simulink model "parameterOptimizerExcavator"  (R2025a)
settings: Solver=ode15s  StartTime=0.0  StopTime=10  RelTol=1e-3
model workspace (MATLAB code in the model file):
  | %% Weights
  | bomWeight = 200.04;
  | stickWeight = 158.71;
  | bucketWeight = 71.311;
  | 
  | %% Cylinders
  | % cylinder One
  | cylinderOneDamping = 1000;
  | cylinderOnePistonCrossSectionalAreaChamberA = 0.1403;
  | cylinderOnePistonCrossSectionalAreaChamberB = 0.17443;
  | cylinderOnePistonStroke = 529.98;
  | cylinderOneDeadVolumeChamberA = 0.04316;
  | cylinderOneDeadVolumeChamberB = 0.054177;
  | 
  | %cylinder Two
  | cylinderTwoDamping = 1000;
  | cylinderTwoPistonCrossSectionalAreaChamberA = 0.18189;
  | cylinderTwoPistonCrossSectionalAreaChamberB = 0.1784;
  | cylinderTwoPistonStroke = 652.71;
  | cylinderTwoDeadVolumeChamberA = 0.036781;
  | cylinderTwoDeadVolumeChamberB = 0.054436;
  | 
  | %% Input
  | inputDelay = 2;
  | 
  | %% Pump
  | %pumpDisplayment = 18;
  | 
  | PGV1 = 0;
  | PGV2 = 10.37811;
  | PGV3 = 21.47722;
  | PGV4 = 32.57634;
  | PGV5 = 43.67545;
  | PGV6 = 54.77457;
  | PGV7 = 65.87369;
  | PGV8 = 76.9728;
  | PGV9 = 88.07192;
  | PGV10 = 99.17103;
  | PGV11 = 110.27015;
  | PGV12 = 121.36926;
  | PGV13 = 132.46838;
  | PGV14 = 143.56749;
  | PGV15 = 154.66661;
  | PGV16 = 165.76572;
  | PGV17 = 176.86484;
  | PGV18 = 187.96396;
  | PGV19 = 199.06307;
  | PGV20 = 210.16219;
  | PGV21 = 221.2613;
  | PGV22 = 232.36042;
  | PGV23 = 243.45953;
  | PGV24 = 254.55865;
  | PGV25 = 265.65776;
  | PGV26 = 276.75688;
  | PGV27 = 287.85599;
  | PGV28 = 298.95511;
  | PGV29 = 310.05422;
  | PGV30 = 321.15334;
  | pumpPressureGainVector = [PGV1 PGV2 PGV3 PGV4 PGV5 PGV6 PGV7 PGV8 PGV9 PGV10 PGV11 PGV12 PGV13 PGV14 PGV15 PGV16 PGV17 PGV18 PGV19 PGV20 PGV21 PGV22 PGV23 PGV24 PGV25 PGV26 PGV27 PGV28 PGV29 PGV30];
  | 
  | SAV1 = 1000;
  | SAV2 = 1200;
  | SAV3 = 1500;
  | SAV4 = 1800;
  | pumpAnglularVelocityVector = [SAV1 SAV2 SAV3 SAV4];
  | 
  | pumpAngluarVelocityThreshold = 10;
  | 
  | %% new pump
  | pumpDisplacement = 0.00013254;
  | pumpNominalShaftAngularVelocity = 116.48;
  | pumpNominalPressureGain = 4.2749;
undefined symbols (not defined in the file): Excavator_Param, X, Y, Z
libraries: sm_lib x65, fl_lib x19, nesl_utility x17, SimscapeFluids_lib x9, simulink_extras x8
(part 1 of 4)
settings Model: Creator=eliasalbag  LastModifiedBy=Viktor Traktor
settings DataIOCC: ReturnWorkspaceOutputsName=SDOSimTest_Log

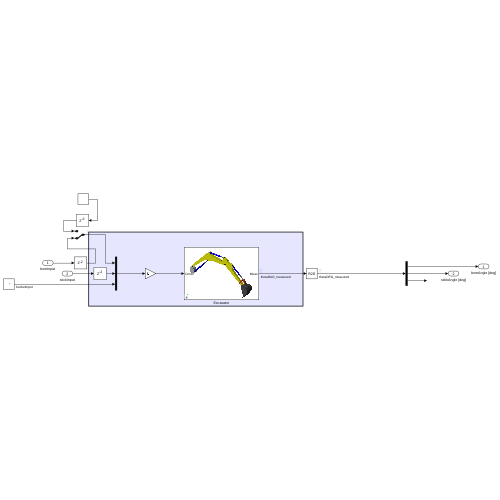
[thumbnail: Simulink's stored preview of the top-level diagram]
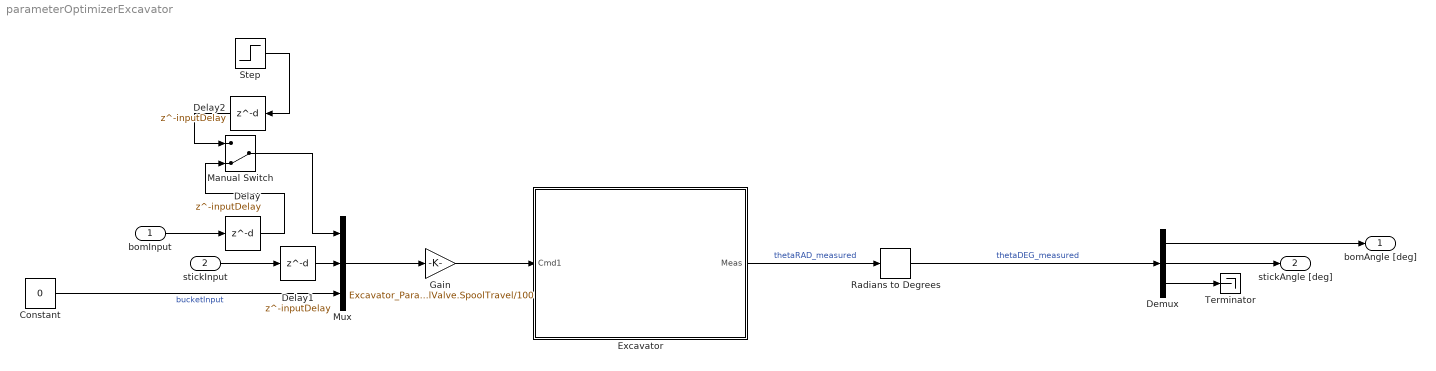
== system parameterOptimizerExcavator ==
  bomInput : Inport
  stickInput : Inport  Port=2
  Constant : Constant  Value=0
  Delay : Delay  DelayLength=inputDelay
  Delay1 : Delay  DelayLength=inputDelay
  Delay2 : Delay  DelayLength=inputDelay
  Demux : Demux  Outputs=3
  Excavator : Subsystem  mask{D=0}
      mask prompts: D "Damping"
      mask Display: image('Skärmbild 2025-05-16 122333.png');
  Gain : Gain  Gain=Excavator_Param.DirectionalValve.SpoolTravel/100
  Manual Switch : ManualSwitch  CurrentSetting=0
  Mux : Mux  Inputs=3
  Radians to Degrees : simulink_extras/Transformations/Radians to Degrees
  Step : Step  After=-100  SampleTime=0.01
  Terminator : Terminator
  bomAngle [deg] : Outport
  stickAngle [deg] : Outport  Port=2
  wires:
  Excavator/1(Meas) -> Radians to Degrees/1  "thetaRAD_measured"
  Mux/1 -> Gain/1
  bomInput/1 -> Delay/1
  Radians to Degrees/1 -> Demux/1  "thetaDEG_measured"
  Constant/1 -> Mux/3  "bucketInput"
  Demux/3 -> Terminator/1
  Demux/2 -> stickAngle [deg]/1
  Demux/1 -> bomAngle [deg]/1
  Gain/1 -> Excavator/1(Cmd1)
  stickInput/1 -> Delay1/1
  Delay/1 -> Manual Switch/2
  Delay1/1 -> Mux/2
  Manual Switch/1 -> Mux/1
  Step/1 -> Delay2/1
  Delay2/1 -> Manual Switch/1

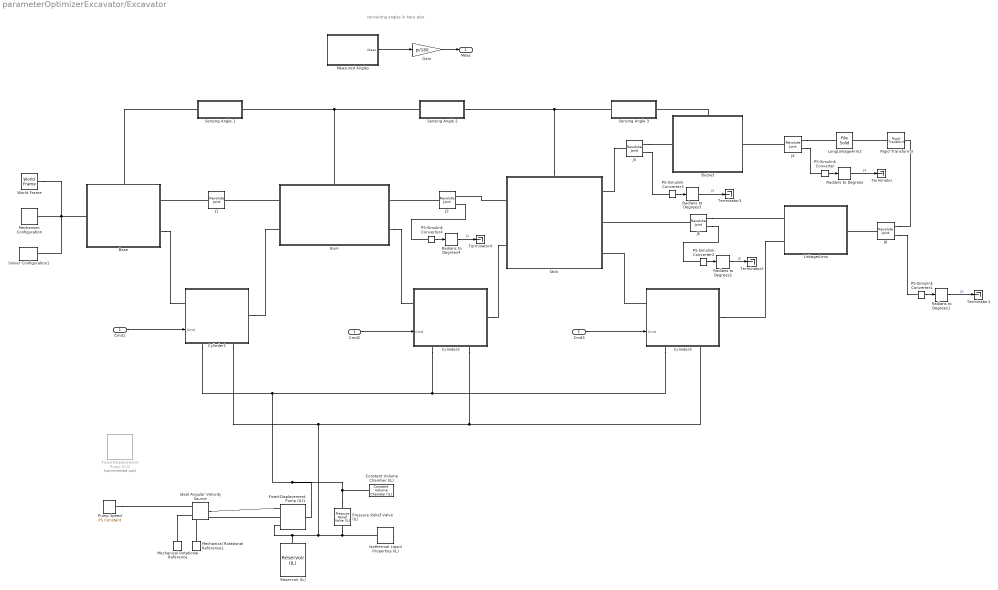
== system parameterOptimizerExcavator/Excavator ==
  note: converting angles in here also
  Cmd1 : Inport
  Base : Subsystem
      settings: PortSchema="{\"entries\":[{\"content\":{\"sides\":[{\"content\":{\"connectorIds\":[\"LConn1\"]},\"type\":\"ConnectorPlacement.EquallySpacedRectSide\",\"uuid\":\"40ecd481-0f87-4ac6-81e7-411d2e7a87dc\"},{\"content\":{\"connectorIds\":[\"RConn1\",\"RConn2\"],\"side\":\"RIGHT\"},\"type\":\"ConnectorPlacement.EquallySpacedRectSide\",\"uuid\":\"4ae56660-704d-4a11-a2e7-42dc450a906f\"},{\"content\":{\"connectorIds\":[\"LConn2\"],\"side\":\"TOP\"},\"type\":\"ConnectorPlacement.EquallySpacedRectSide\",\"uuid\":\"88ba4c47-909e-475c-98b2-d2ec55f2c628\"}]},\"type\":\"ConnectorPlacement.EquallySpacedConnector\",\"uuid\":\"875afadf-353a-4577-a20f-50c01c00738f\"}],\"packageUris\":[\"http://schema.mathworks.com/mf0/Connector/R2020b\"],\"version\":\"1.0\"}"
      mask Display: image('Skärmbild 2025-04-30 163637.png');
  Bom : Subsystem
      settings: PortSchema="{\"entries\":[{\"content\":{\"sides\":[{\"content\":{\"connectorIds\":[\"LConn1\",\"LConn2\"]},\"type\":\"ConnectorPlacement.EquallySpacedRectSide\",\"uuid\":\"7ad98941-c155-4b77-821c-441aa02f495c\"},{\"content\":{\"connectorIds\":[\"RConn1\",\"RConn2\"],\"side\":\"RIGHT\"},\"type\":\"ConnectorPlacement.EquallySpacedRectSide\",\"uuid\":\"f5fb3b40-b535-47bd-a749-2c1f436a2cdb\"},{\"content\":{\"connectorIds\":[\"LConn3\"],\"side\":\"TOP\"},\"type\":\"ConnectorPlacement.EquallySpacedRectSide\",\"uuid\":\"726e9b82-bc1f-498c-98b8-155d9f00309d\"}]},\"type\":\"ConnectorPlacement.EquallySpacedConnector\",\"uuid\":\"e0155be9-0ff1-4a5f-ae8d-a122aa83cbac\"}],\"packageUris\":[\"http://schema.mathworks.com/mf0/Connector/R2020b\"],\"version\":\"1.0\"}"
      mask Display: image('Skärmbild 2025-05-01 094232.png');
  Bucket : Subsystem
      settings: PortSchema="{\"entries\":[{\"content\":{\"sides\":[{\"content\":{\"connectorIds\":[\"LConn1\"]},\"type\":\"ConnectorPlacement.EquallySpacedRectSide\",\"uuid\":\"5de28302-4101-44f3-9c23-279c450fdd15\"},{\"content\":{\"connectorIds\":[\"RConn1\"],\"side\":\"RIGHT\"},\"type\":\"ConnectorPlacement.EquallySpacedRectSide\",\"uuid\":\"b0db8830-510e-47ef-9140-b2643c0c8376\"},{\"content\":{\"connectorIds\":[\"LConn2\"],\"side\":\"TOP\"},\"type\":\"ConnectorPlacement.EquallySpacedRectSide\",\"uuid\":\"09d89f5e-8f1e-4430-8208-03f2526c5b85\"}]},\"type\":\"ConnectorPlacement.EquallySpacedConnector\",\"uuid\":\"9e049277-2e17-4388-a3ed-55a7f1fde4cc\"}],\"packageUris\":[\"http://schema.mathworks.com/mf0/Connector/R2020b\"],\"version\":\"1.0\"}"
      mask Display: image('Skärmbild 2025-05-02 202436.png');
  Cmd2 : InportShadow
  Cmd3 : InportShadow
  Constant Volume Chamber (IL) : fl_lib/Isothermal Liquid/Elements/Constant Volume Chamber (IL)  volume=1e-4 m^3  p_I_specify=off  p_I_priority=High  p_I=0.101325 MPa  p_I_nominal_specify=off  p_I_nominal_value=1  p_I_nominal_unit=MPa
      settings: InternalSimscapePortConfiguration="{\"Bottom\":[],\"Left\":[{\"id\":\"A\",\"label\":\"A\",\"type\":\"foundation.isothermal_liquid.isothermal_liquid\"}],\"Right\":[],\"Top\":[]}"
  Cylinder1 : Subsystem
      settings: PortSchema="{\"entries\":[{\"content\":{\"sides\":[{\"content\":{\"connectorIds\":[\"LConn1\",\"In1\"]},\"type\":\"ConnectorPlacement.EquallySpacedRectSide\",\"uuid\":\"958c3393-df8d-4c6f-89df-92ae8f6a338c\"},{\"content\":{\"connectorIds\":[\"RConn1\"],\"side\":\"RIGHT\"},\"type\":\"ConnectorPlacement.EquallySpacedRectSide\",\"uuid\":\"7fbd6d33-fc32-41eb-a764-fc12f800bd43\"},{\"content\":{\"side\":\"TOP\"},\"type\":\"ConnectorPlacement.EquallySpacedRectSide\",\"uuid\":\"2a2fac5b-7b8e-4bd5-9693-24b32f9ec475\"},{\"content\":{\"connectorIds\":[\"RConn2\",\"RConn3\"],\"side\":\"BOTTOM\"},\"type\":\"ConnectorPlacement.EquallySpacedRectSide\",\"uuid\":\"152fac46-1909-43ca-b282-7d5220c5a160\"}]},\"type\":\"ConnectorPlacement.EquallySpacedConnector\",\"uuid\":\"942b4f77-d0ef-4ef4-96e1-eaf5fcd20a12\"}],\"packageUris\":[\"http://schema.mathworks.com/mf0/Connector/R2020b\"],\"version\":\"1.0\"}"
      mask Display: image('Skärmbild 2025-05-02 202508.png');
  Cylinder2 : Subsystem
      settings: PortSchema="{\"entries\":[{\"content\":{\"sides\":[{\"content\":{\"connectorIds\":[\"LConn1\",\"In1\"]},\"type\":\"ConnectorPlacement.EquallySpacedRectSide\",\"uuid\":\"57f8ce67-ce53-4554-827a-ade4073837f1\"},{\"content\":{\"connectorIds\":[\"RConn1\"],\"side\":\"RIGHT\"},\"type\":\"ConnectorPlacement.EquallySpacedRectSide\",\"uuid\":\"2d7b50e6-8862-4672-bf86-700cfda39af2\"},{\"content\":{\"side\":\"TOP\"},\"type\":\"ConnectorPlacement.EquallySpacedRectSide\",\"uuid\":\"6448b736-3558-4b72-a3be-02cdc9d0d1c5\"},{\"content\":{\"connectorIds\":[\"RConn2\",\"RConn3\"],\"side\":\"BOTTOM\"},\"type\":\"ConnectorPlacement.EquallySpacedRectSide\",\"uuid\":\"d65b4c05-b673-4eae-8b65-2a19aca8236c\"}]},\"type\":\"ConnectorPlacement.EquallySpacedConnector\",\"uuid\":\"43cefb1d-1bfc-4d29-867b-e7529d2d57fb\"}],\"packageUris\":[\"http://schema.mathworks.com/mf0/Connector/R2020b\"],\"version\":\"1.0\"}"
      mask Display: image('Skärmbild 2025-05-02 202508.png');
  Cylinder3 : Subsystem
      settings: PortSchema="{\"entries\":[{\"content\":{\"sides\":[{\"content\":{\"connectorIds\":[\"LConn1\",\"In1\"]},\"type\":\"ConnectorPlacement.EquallySpacedRectSide\",\"uuid\":\"57f8ce67-ce53-4554-827a-ade4073837f1\"},{\"content\":{\"connectorIds\":[\"RConn1\"],\"side\":\"RIGHT\"},\"type\":\"ConnectorPlacement.EquallySpacedRectSide\",\"uuid\":\"2d7b50e6-8862-4672-bf86-700cfda39af2\"},{\"content\":{\"side\":\"TOP\"},\"type\":\"ConnectorPlacement.EquallySpacedRectSide\",\"uuid\":\"6448b736-3558-4b72-a3be-02cdc9d0d1c5\"},{\"content\":{\"connectorIds\":[\"RConn2\",\"RConn3\"],\"side\":\"BOTTOM\"},\"type\":\"ConnectorPlacement.EquallySpacedRectSide\",\"uuid\":\"3b9bbe70-3b78-4081-87f5-0faddfe5faea\"}]},\"type\":\"ConnectorPlacement.EquallySpacedConnector\",\"uuid\":\"43cefb1d-1bfc-4d29-867b-e7529d2d57fb\"}],\"packageUris\":[\"http://schema.mathworks.com/mf0/Connector/R2020b\"],\"version\":\"1.0\"}"
      mask Display: image('Skärmbild 2025-05-02 202508.png');
  Fixed-Displacement Pump (IL)1 : SimscapeFluids_lib/Isothermal Liquid/Pumps & Motors/Fixed-Displacement Pump (IL)  leakage_friction_spec=fluids.isothermal_liquid.pumps_motors.enum.pump_motor_loss_spec.analytical  displacement=pumpDisplacement m^3/rad  omega_nominal=pumpNominalShaftAngularVelocity rad/s  p_nominal=pumpNominalPressureGain MPa  vol_eff_nominal=0.92  mech_eff_nominal=0.88  no_load_torque=0 N*m  p_diff_eff_TLU=[.1, 1, 2] MPa  omega_eff_TLU=[250, 500, 1000, 2000, 3000, 4000] rpm  vol_eff_TLU=[.816, .908, .954, .977, .981, .984; .325, .663, .831, .916, .925, .946; .137, .568, .78, .892, .893, .91]  mech_eff_TLU=[.996, .996, .996, .996, .996, .996; .988, .989, .989, .989, .989, .99; .981, .981, .982, .982, .983, .984]  p_diff_loss_TLU=[.1, 1, 2] MPa  omega_loss_TLU=[250, 500, 1000, 2000, 3000, 4000] rpm  vol_loss_TLU=1e-3 * [.023, .023, .023, .023, .0285, .032; .0844, .0842, .0845, .084, .1125, .108; .1079, .108, .11, .108, .1605, .18] m^3/s  mech_loss_TLU=[.002, .002, .002, .002, .002, .002; .0607, .0556, .0556, .0556, .0556, .0505; .1937, .1937, .1833, .1833, .1729, .1626] N*m  vol_eff_min=1e-3  vol_eff_max=1  mech_eff_min=1e-3  mech_eff_max=1  pressure_threshold=1e-3 MPa  omega_threshold=100 rpm  supplied_range_check=simscape.enum.assert.action.none  pump_mode_check=simscape.enum.assert.action.none  pressure_check=simscape.enum.assert.action.none  p_min_valid=0.101325 MPa
      settings: InternalSimscapePortConfiguration="{\"Bottom\":[{\"id\":\"A\",\"label\":\"A\",\"type\":\"foundation.isothermal_liquid.isothermal_liquid\"}],\"Left\":[],\"Right\":[{\"id\":\"R\",\"label\":\"R\",\"type\":\"foundation.mechanical.rotational.rotational\"},{\"id\":\"C\",\"label\":\"C\",\"type\":\"foundation.mechanical.rotational.rotational\"}],\"Top\":[{\"id\":\"B\",\"label\":\"B\",\"type\":\"foundation.isothermal_liquid.isothermal_liquid\"}]}"
  Fixed-Displacement Pump (IL)2 : SimscapeFluids_lib/Isothermal Liquid/Pumps & Motors/Fixed-Displacement Pump (IL)  Commented=on  PartSpecification="{\"CollectionId\":\"SimscapeFluids\",\"CollectionVersion\":\"1.0.0\",\"DatasetId\":\"Eaton|PVM:018|simscape.fluids.isothermalLiquid.fixedDisplacementPump\",\"DisplayName\":\"Eaton:PVM:018\"}"  leakage_friction_spec=fluids.isothermal_liquid.pumps_motors.enum.pump_motor_loss_spec.table_efficiency  displacement=pumpDisplayment cm^3/rev  omega_nominal=1800 % Parameter not set rpm  p_nominal=10 % Parameter not set MPa  vol_eff_nominal=0.92 % Parameter not set  mech_eff_nominal=0.88 % Parameter not set  no_load_torque=0 % Parameter not set N*m  p_diff_eff_TLU=pumpPressureGainVector bar  omega_eff_TLU=pumpAnglularVelocityVector rpm  vol_eff_TLU=[0.9933773 0.9986255 1 1;0.9908815 0.9970227 0.9988015 0.9986391;0.9882123 0.9953086 0.9972361 0.9971836;0.9855432 0.9935944 0.9956708 0.9957282;0.982874 0.9918803 0.9941054 0.9942727;0.9809628 0.9901046 0.9924794 0.992827;0.9800522 0.9882469 0.9908036 0.991394;0.9791415 0.9863891 0.9891279 0.989961;0.9782309 0.9845314 0.9874521 0.988528;0.9773202 0.9826736 0.9857764 0.987095;0.9763834 0.9808159 0.984196 0.9858236;0.9754406 0.9789581 0.9826224 0.9845647;0.9744978 0.9771004 0.9810489 0.9833058;0.973555 0.9752426 0.9794753 0.9820468;0.9722953 0.9733813 0.9778456 0.9807183;0.9704577 0.9715138 0.9761613 0.9792853;0.9686202 0.9696463 0.9744771 0.9778523;0.9667827 0.9677789 0.9727928 0.9764193;0.9649452 0.9659114 0.9711086 0.9749863;0.9633236 0.9640355 0.9698474 0.9737089;0.9617784 0.9621582 0.9686255 0.97245;0.9602331 0.9602809 0.9674035 0.9711911;0.9586878 0.9584036 0.9661816 0.9699321;0.9563057 0.9564651 0.9651295 0.9682414;0.9524066 0.9544264 0.9642731 0.9658002;0.9485075 0.9523877 0.9634167 0.9633591;0.9446085 0.950349 0.9625603 0.9609179;0.9407094 0.9483103 0.9617039 0.9584767;0.9360576 0.9469113 0.9607892 0.9566098;0.931177 0.9456055 0.9598677 0.9548364] % Datasheet derived  mech_eff_TLU=[0.001 0.001 0.01192 0.001;0.54982 0.55826 0.52817 0.51523;0.7457 0.73749 0.72894 0.7104;0.82552 0.81697 0.8091 0.79478;0.86515 0.8517 0.84128 0.83826;0.89161 0.87592 0.86458 0.86826;0.89855 0.8853 0.87936 0.88694;0.9055 0.89471 0.89419 0.90566;0.91246 0.90416 0.90907 0.91532;0.91943 0.91365 0.91743 0.92476;0.92432 0.92008 0.92338 0.92926;0.92874 0.9261 0.92933 0.93321;0.93316 0.93215 0.9353 0.93716;0.93759 0.93822 0.94128 0.94113;0.94083 0.94329 0.94509 0.94404;0.94196 0.94674 0.94701 0.94533;0.94308 0.9502 0.94893 0.94662;0.94421 0.95368 0.95086 0.94792;0.94534 0.95717 0.9528 0.94922;0.94547 0.95801 0.95262 0.94983;0.94521 0.95819 0.95216 0.95032;0.94494 0.95838 0.9517 0.95082;0.94468 0.95857 0.95124 0.95132;0.94485 0.95778 0.9502 0.95201;0.94566 0.95552 0.9485 0.95304;0.9444 0.95324 0.94681 0.95407;0.94245 0.95096 0.94511 0.9551;0.9405 0.94866 0.94341 0.95614;0.94063 0.94494 0.94137 0.95543;0.94151 0.941 0.93927 0.95443] % Datasheet derived  p_diff_loss_TLU=[.1, 1, 2] % Parameter not set MPa  omega_loss_TLU=[250, 500, 1000, 2000, 3000, 4000] % Parameter not set rpm  vol_loss_TLU=1e-3 * [.023, .023, .023, .023, .0285, .032; .0844, .0842, .0845, .084, .1125, .108; .1079, .108, .11, .108, .1605, .18] % Parameter not set m^3/s  mech_loss_TLU=[.002, .002, .002, .002, .002, .002; .0607, .0556, .0556, .0556, .0556, .0505; .1937, .1937, .1833, .1833, .1729, .1626] % Parameter not set N*m  vol_eff_min=1e-3 % Parameter not set  vol_eff_max=1 % Parameter not set  mech_eff_min=1e-3 % Parameter not set  mech_eff_max=1 % Parameter not set  pressure_threshold=0.001 % Library default MPa  omega_threshold=pumpAngluarVelocityThreshold rpm  supplied_range_check=simscape.enum.assert.action.none  pump_mode_check=simscape.enum.assert.action.none  pressure_check=simscape.enum.assert.action.none  p_min_valid=0.101325 % Parameter not set MPa
      settings: AttributesFormatString=Eaton:PVM:018  InternalSimscapePortConfiguration="{\"Bottom\":[{\"id\":\"A\",\"label\":\"A\",\"type\":\"foundation.isothermal_liquid.isothermal_liquid\"}],\"Left\":[],\"Right\":[{\"id\":\"R\",\"label\":\"R\",\"type\":\"foundation.mechanical.rotational.rotational\"},{\"id\":\"C\",\"label\":\"C\",\"type\":\"foundation.mechanical.rotational.rotational\"}],\"Top\":[{\"id\":\"B\",\"label\":\"B\",\"type\":\"foundation.isothermal_liquid.isothermal_liquid\"}]}"
  Gain : Gain  Gain=pi/180
  Ideal Angular Velocity Source : fl_lib/Mechanical/Mechanical Sources/Ideal Angular Velocity Source
  Isothermal Liquid Properties (IL) : fl_lib/Isothermal Liquid/Utilities/Isothermal Liquid Properties (IL)  rho_L_atm=845 kg/m^3  bulk_modulus_model=foundation.enum.bulk_modulus_model.const  beta_gain=6  beta_L_atm=1.59e9 Pa  nu_atm=52.63 cSt  p_atm=0.101325 MPa  p_min=1 Pa  properties_range_check=simscape.enum.assert.action.error  air_fraction=0.004  polytropic_index=1.0  rho_g_atm=1.225 kg/m^3  air_dissolution_model=false  p_crit=3 MPa
  J1 : sm_lib/Joints/Revolute Joint  JointMode=Normal  CompositeWrenchDir=FollowerOnBase  CompositeWrenchFrame=BaseFrame  SenseConstraintForce=off  SenseConstraintTorque=off  SenseTotalForce=off  SenseTotalTorque=off  PositionTargetSpecify=on  PositionTargetPriority=Low  PositionTargetValue=0  PositionTargetValueUnits=deg  VelocityTargetSpecify=off  VelocityTargetPriority=High  VelocityTargetValue=0  VelocityTargetValueUnits=deg/s  EquilibriumPosition=0  EquilibriumPositionUnits=deg  SpringStiffness=0  SpringStiffnessUnits=N*m/deg  DampingCoefficient=Excavator_Param.Joint1.Damping  DampingCoefficientUnits=N*m/(deg/s)  LowerLimitSpecify=off  LowerLimitBound=-15  LowerLimitBoundUnits=deg  LowerLimitStiffness=1e5  LowerLimitStiffnessUnits=N*m/deg  LowerLimitDamping=10  LowerLimitDampingUnits=N*m/(deg/s)  LowerLimitTransitionRegionWidth=1  LowerLimitTransitionRegionWidthUnits=deg  UpperLimitSpecify=off  UpperLimitBound=15  UpperLimitBoundUnits=deg  UpperLimitStiffness=1e5  UpperLimitStiffnessUnits=N*m/deg  UpperLimitDamping=10  UpperLimitDampingUnits=N*m/(deg/s)  UpperLimitTransitionRegionWidth=1  UpperLimitTransitionRegionWidthUnits=deg  TorqueActuationMode=NoTorque  MotionActuationMode=ComputedMotion  SensePosition=off  SenseVelocity=off  SenseAcceleration=off  SenseTorqueForce=off  SenseLowerLimitTorqueForce=off  SenseUpperLimitTorqueForce=off
  J2 : sm_lib/Joints/Revolute Joint  JointMode=Normal  CompositeWrenchDir=FollowerOnBase  CompositeWrenchFrame=BaseFrame  SenseConstraintForce=off  SenseConstraintTorque=off  SenseTotalForce=off  SenseTotalTorque=off  PositionTargetSpecify=on  PositionTargetPriority=Low  PositionTargetValue=0  PositionTargetValueUnits=deg  VelocityTargetSpecify=off  VelocityTargetPriority=High  VelocityTargetValue=0  VelocityTargetValueUnits=deg/s  EquilibriumPosition=0  EquilibriumPositionUnits=deg  SpringStiffness=0  SpringStiffnessUnits=N*m/deg  DampingCoefficient=Excavator_Param.Joint2.Damping  DampingCoefficientUnits=N*m/(deg/s)  LowerLimitSpecify=off  LowerLimitBound=-90  LowerLimitBoundUnits=deg  LowerLimitStiffness=1e4  LowerLimitStiffnessUnits=N*m/deg  LowerLimitDamping=10  LowerLimitDampingUnits=N*m/(deg/s)  LowerLimitTransitionRegionWidth=0.1  LowerLimitTransitionRegionWidthUnits=deg  UpperLimitSpecify=on  UpperLimitBound=26  UpperLimitBoundUnits=deg  UpperLimitStiffness=1e20  UpperLimitStiffnessUnits=N*m/deg  UpperLimitDamping=1e12  UpperLimitDampingUnits=N*m/(deg/s)  UpperLimitTransitionRegionWidth=0.1  UpperLimitTransitionRegionWidthUnits=deg  TorqueActuationMode=NoTorque  MotionActuationMode=ComputedMotion  SensePosition=on  SenseVelocity=off  SenseAcceleration=off  SenseTorqueForce=off  SenseLowerLimitTorqueForce=off  SenseUpperLimitTorqueForce=off
  J3 : sm_lib/Joints/Revolute Joint  JointMode=Normal  CompositeWrenchDir=FollowerOnBase  CompositeWrenchFrame=BaseFrame  SenseConstraintForce=off  SenseConstraintTorque=off  SenseTotalForce=off  SenseTotalTorque=off  PositionTargetSpecify=off  PositionTargetPriority=High  PositionTargetValue=0  PositionTargetValueUnits=deg  VelocityTargetSpecify=off  VelocityTargetPriority=High  VelocityTargetValue=0  VelocityTargetValueUnits=deg/s  EquilibriumPosition=0  EquilibriumPositionUnits=deg  SpringStiffness=0  SpringStiffnessUnits=N*m/deg  DampingCoefficient=100  DampingCoefficientUnits=N*m/(deg/s)  LowerLimitSpecify=off  LowerLimitBound=-90  LowerLimitBoundUnits=deg  LowerLimitStiffness=1e4  LowerLimitStiffnessUnits=N*m/deg  LowerLimitDamping=10  LowerLimitDampingUnits=N*m/(deg/s)  LowerLimitTransitionRegionWidth=0.1  LowerLimitTransitionRegionWidthUnits=deg  UpperLimitSpecify=off  UpperLimitBound=90  UpperLimitBoundUnits=deg  UpperLimitStiffness=1e4  UpperLimitStiffnessUnits=N*m/deg  UpperLimitDamping=10  UpperLimitDampingUnits=N*m/(deg/s)  UpperLimitTransitionRegionWidth=0.1  UpperLimitTransitionRegionWidthUnits=deg  TorqueActuationMode=NoTorque  MotionActuationMode=ComputedMotion  SensePosition=on  SenseVelocity=off  SenseAcceleration=off  SenseTorqueForce=off  SenseLowerLimitTorqueForce=off  SenseUpperLimitTorqueForce=off
  J4 : sm_lib/Joints/Revolute Joint  JointMode=Normal  CompositeWrenchDir=FollowerOnBase  CompositeWrenchFrame=BaseFrame  SenseConstraintForce=off  SenseConstraintTorque=off  SenseTotalForce=off  SenseTotalTorque=off  PositionTargetSpecify=off  PositionTargetPriority=High  PositionTargetValue=0  PositionTargetValueUnits=deg  VelocityTargetSpecify=off  VelocityTargetPriority=High  VelocityTargetValue=0  VelocityTargetValueUnits=deg/s  EquilibriumPosition=0  EquilibriumPositionUnits=deg  SpringStiffness=0  SpringStiffnessUnits=N*m/deg  DampingCoefficient=100  DampingCoefficientUnits=N*m/(deg/s)  LowerLimitSpecify=off  LowerLimitBound=-90  LowerLimitBoundUnits=deg  LowerLimitStiffness=1e4  LowerLimitStiffnessUnits=N*m/deg  LowerLimitDamping=10  LowerLimitDampingUnits=N*m/(deg/s)  LowerLimitTransitionRegionWidth=0.1  LowerLimitTransitionRegionWidthUnits=deg  UpperLimitSpecify=off  UpperLimitBound=90  UpperLimitBoundUnits=deg  UpperLimitStiffness=1e4  UpperLimitStiffnessUnits=N*m/deg  UpperLimitDamping=10  UpperLimitDampingUnits=N*m/(deg/s)  UpperLimitTransitionRegionWidth=0.1  UpperLimitTransitionRegionWidthUnits=deg  TorqueActuationMode=NoTorque  MotionActuationMode=ComputedMotion  SensePosition=on  SenseVelocity=off  SenseAcceleration=off  SenseTorqueForce=off  SenseLowerLimitTorqueForce=off  SenseUpperLimitTorqueForce=off
  J5 : sm_lib/Joints/Revolute Joint  JointMode=Normal  CompositeWrenchDir=FollowerOnBase  CompositeWrenchFrame=BaseFrame  SenseConstraintForce=off  SenseConstraintTorque=off  SenseTotalForce=off  SenseTotalTorque=off  PositionTargetSpecify=off  PositionTargetPriority=High  PositionTargetValue=0  PositionTargetValueUnits=deg  VelocityTargetSpecify=off  VelocityTargetPriority=High  VelocityTargetValue=0  VelocityTargetValueUnits=deg/s  EquilibriumPosition=0  EquilibriumPositionUnits=deg  SpringStiffness=0  SpringStiffnessUnits=N*m/deg  DampingCoefficient=100  DampingCoefficientUnits=N*m/(deg/s)  LowerLimitSpecify=off  LowerLimitBound=-90  LowerLimitBoundUnits=deg  LowerLimitStiffness=1e4  LowerLimitStiffnessUnits=N*m/deg  LowerLimitDamping=10  LowerLimitDampingUnits=N*m/(deg/s)  LowerLimitTransitionRegionWidth=0.1  LowerLimitTransitionRegionWidthUnits=deg  UpperLimitSpecify=off  UpperLimitBound=90  UpperLimitBoundUnits=deg  UpperLimitStiffness=1e4  UpperLimitStiffnessUnits=N*m/deg  UpperLimitDamping=10  UpperLimitDampingUnits=N*m/(deg/s)  UpperLimitTransitionRegionWidth=0.1  UpperLimitTransitionRegionWidthUnits=deg  TorqueActuationMode=NoTorque  MotionActuationMode=ComputedMotion  SensePosition=on  SenseVelocity=off  SenseAcceleration=off  SenseTorqueForce=off  SenseLowerLimitTorqueForce=off  SenseUpperLimitTorqueForce=off
  J6 : sm_lib/Joints/Revolute Joint  JointMode=Normal  CompositeWrenchDir=FollowerOnBase  CompositeWrenchFrame=BaseFrame  SenseConstraintForce=off  SenseConstraintTorque=off  SenseTotalForce=off  SenseTotalTorque=off  PositionTargetSpecify=on  PositionTargetPriority=Low  PositionTargetValue=-70  PositionTargetValueUnits=deg  VelocityTargetSpecify=off  VelocityTargetPriority=High  VelocityTargetValue=0  VelocityTargetValueUnits=deg/s  EquilibriumPosition=0  EquilibriumPositionUnits=deg  SpringStiffness=0  SpringStiffnessUnits=N*m/deg  DampingCoefficient=100  DampingCoefficientUnits=N*m/(deg/s)  LowerLimitSpecify=on  LowerLimitBound=-120  LowerLimitBoundUnits=deg  LowerLimitStiffness=1e4  LowerLimitStiffnessUnits=N*m/deg  LowerLimitDamping=10  LowerLimitDampingUnits=N*m/(deg/s)  LowerLimitTransitionRegionWidth=0.1  LowerLimitTransitionRegionWidthUnits=deg  UpperLimitSpecify=on  UpperLimitBound=-30  UpperLimitBoundUnits=deg  UpperLimitStiffness=1e4  UpperLimitStiffnessUnits=N*m/deg  UpperLimitDamping=10  UpperLimitDampingUnits=N*m/(deg/s)  UpperLimitTransitionRegionWidth=0.1  UpperLimitTransitionRegionWidthUnits=deg  TorqueActuationMode=NoTorque  MotionActuationMode=ComputedMotion  SensePosition=on  SenseVelocity=off  SenseAcceleration=off  SenseTorqueForce=off  SenseLowerLimitTorqueForce=off  SenseUpperLimitTorqueForce=off
  LinkageArms : Subsystem
      mask Display: image('Skärmbild 2025-05-02 202545.png');
  LongLinkageArm2 : sm_lib/Body Elements/File Solid  ExtGeomFileName=CAD/STEPfiles/Lankarm_langCut.stp  UnitType=Custom  ExtGeomFileUnits=mm  StepReaderType=HEX  ExportConvexHullGeometry=off  InertiaType=CalculateFromGeometry  BasedOnType=Density  Density=1000  DensityUnits=kg/m^3  Mass=1  MassUnits=kg  CenterOfMass=[0 0 0]  CenterOfMassUnits=m  MomentsOfInertia=[1 1 1]  MomentsOfInertiaUnits=kg*m^2  ProductsOfInertia=[0 0 0]  ProductsOfInertiaUnits=kg*m^2  GraphicType=FromGeometry  MarkerShape=Sphere  MarkerSize=10  GraphicVisPropType=SimpleVisualProperties  GraphicDiffuseColor=[0.851 0.3255 0.09804]  GraphicOpacity=1  GraphicSpecularColor=[0.5 0.5 0.5 1.0]  GraphicAmbientColor=[0.15 0.15 0.15 1.0]  GraphicEmissiveColor=[0.0 0.0 0.0 1.0]  GraphicShininess=75  DoExposeReferenceFrame=off  SerializedFrames=<Frames><Frame><Id>Frame1</Id><Value><Name>F1</Name><Origin><Source>GeometricFeature</Source><FeatureName>cylindrical surface 69</FeatureName></Origin><PrimaryAxis><DefinedDirection>-Y</DefinedDirection><Source>ReferenceFrame</Source><SourceDirection>+Y</SourceDirection><FeatureName></FeatureName></PrimaryAxis><SecondaryAxis><DefinedDirection>+X</DefinedDirection><Source>ReferenceFrame</Source><SourceDirection>+Z</SourceDirection><FeatureName></FeatureName></SecondaryAxis></Value></Frame><Frame><Id>Frame2</Id><Value><Name>F2</Name><Origin><Source>GeometricFeature</Source><FeatureName>cylindrical surface 70</FeatureName></Origin><PrimaryAxis><DefinedDirection>-Y</DefinedDirection><Source>ReferenceFrame</Source><SourceDirection>+Y</SourceDirection><FeatureName></FeatureName></PrimaryAxis><SecondaryAxis><DefinedDirection>+X</DefinedDirection><Source>ReferenceFrame</Source><SourceDirection>+Z</SourceDirection><FeatureName></FeatureName></SecondaryAxis></Value></Frame></Frames>
  Measured Angles : Subsystem
  Mechanical Rotational Reference : fl_lib/Mechanical/Rotational Elements/Mechanical Rotational Reference
  Mechanical Rotational Reference1 : fl_lib/Mechanical/Rotational Elements/Mechanical Rotational Reference
  Mechanism Configuration : sm_lib/Utilities/Mechanism Configuration  UniformGravity=Constant  GravityVector=[0 -9.82 0]  GravityVectorUnits=m/s^2  LinearizationDelta=0.001  JointModeTransitionNonlinearIterations=2
  PS-Simulink Converter{,1..4} (5 alike) : nesl_utility/PS-Simulink Converter  PhysicalDomain=network_engine_domain  SubClassName=ps_output  LeftPortType=input  RightPortType=output  PseudoPeriodic=off  Frequencies=[]  VectorFormat=inherit  Unit=rad  AffineConversion=off
  Pressure Relief Valve (IL) : SimscapeFluids_lib/Isothermal Liquid/Valves & Orifices/Pressure Control Valves/Pressure Relief Valve (IL)  set_pressure_spec=foundation.enum.constant_controlled.constant  opening_spec=fluids.isothermal_liquid.valves_orifices.enum.PressureOpeningSpec.Linear  pressure_spec=fluids.isothermal_liquid.valves_orifices.enum.pressure_control_spec.dp  p_set_gauge=0.1 MPa  p_set_differential=27579000 Pa  p_range=2757900 Pa  area_max=0.002 m^2  area_leak=1e-9 m^2  p_diff_TLU=[0.2 : 0.2 : 1.2] MPa  p_gauge_TLU=[0.2 : 0.2 : 1.2] MPa  valve_area_TLU=[1e-10, 2e-06, 4e-06, 6e-06, 8e-06, 1e-05] m^2  vol_flow_TLU=[1e-09, 3.6e-05, 8.9e-05, .00015, .00023, .00031] m^3/s  area=inf m^2  Cd=0.7  Re_c=12  smoothing_factor=0  pressure_recovery=false  opening_dynamics=false  tau=0.1 s
      settings: InternalSimscapePortConfiguration="{\"Bottom\":[],\"Left\":[{\"id\":\"A\",\"label\":\"A\",\"type\":\"foundation.isothermal_liquid.isothermal_liquid\"}],\"Right\":[{\"id\":\"B\",\"label\":\"B\",\"type\":\"foundation.isothermal_liquid.isothermal_liquid\"}],\"Top\":[]}"
  Pump Speed : fl_lib/Physical Signals/Sources/PS Constant  constant=150
  Radians to Degrees{,1..4} (5 alike) : simulink_extras/Transformations/Radians to Degrees
  Reservoir (IL) : fl_lib/Isothermal Liquid/Elements/Reservoir (IL)  reservoir_type=foundation.enum.constant_controlled.constant  pressure_spec=foundation.enum.pressure_spec.atmospheric  reservoir_pressure=0.101325 MPa
  Rigid Transform3 : sm_lib/Frames and Transforms/Rigid Transform  RotationMethod=None  FollAlignAxisA=+X  BaseAlignAxisA=+Y  FollAlignAxisB=+Y  BaseAlignAxisB=+Z  RotationStandardAxis=+Z  RotationAngle=0  RotationAngleUnits=deg  RotationArbitraryAxis=[0 0 1]  RotationSequenceAxes=FollowerAxes  RotationSequence=XYX  RotationSequenceAngles=[0 0 0]  RotationSequenceAnglesUnits=deg  RotationMatrix=[1 0 0;0 1 0;0 0 1]  Quaternion=[1 0 0 0]  TranslationMethod=StandardAxis  TranslationCartesianOffset=[0 0 0]  TranslationCartesianOffsetUnits=m  TranslationStandardAxis=-Z  TranslationStandardOffset=-(Excavator_Param.LinkageArmLong.CutoutWidth/2) + (Excavator_Param.Stick.Width/2)  TranslationStandardOffsetUnits=m  TranslationROffset=0  TranslationROffsetUnits=m  TranslationThetaOffset=0  TranslationThetaOffsetUnits=deg  TranslationZOffset=0  TranslationZOffsetUnits=m
  Sensing Angle 1 : Subsystem
  Sensing Angle 2 : Subsystem
  Sensing Angle 3 : Subsystem
  Solver Configuration1 : nesl_utility/Solver Configuration  PhysicalDomain=network_engine_domain  SubClassName=solver  LeftPortType=input  RightPortType=generic  Tones=[]  Harmonics=[]  SimulateNoise=off  Profile=off  UseLocalSampling=off  EnableSwitchedLinearOptims=on  FrequencyDomain=off  UseCCode=off  RelTol=0.001  AbsTol=0.001  MinStep=1e-09  ToWorkspace=off  RevertToSquareIcSolve=off  NumHomotopyIterations=100  PhasorMode=off  PhasorModeNumHarmonics=1  ConsistencySolver=NEWTON_XTOL_AFTER_FTOL  IndexReductionMethod=DerivativeReplacement  DoDC=off  ResidualTolerance=1e-09  ConsistencyTolSource=GLOBAL  ConsistencyAbsTol=0.001  ConsistencyRelTol=0.001  ConsistencyTolFactor=0.001  UseLocalSolver=off  LocalSolverChoice=NE_BACKWARD_EULER_ADVANCER  ResolveIndetEquations=on  FunctionEvalNumThread=1  LocalSolverSampleTime=0.001  DoFixedCost=off  MaxNonlinIter=3  MaxModeIter=2  ComputeImpulses=off  ImpulseIterations=2  LinearAlgebra=Sparse  LinearAlgebraNumThread=0  EquationFormulation=NE_TIME_EF  DelaysMemoryBudget=1024  AutomaticFiltering=on  FilteringTimeConstant=0.001  PartitionStorageMethod=AS_NEEDED  PartitionMemoryBudget=1024  PartitionMethod=ROBUST  MultibodyUseLocalSolver=off  MultibodyLocalSolverChoice=ODE1  MultibodyLocalSolverSampleTime=0.001
  Stick : Subsystem
      settings: PortSchema="{\"entries\":[{\"content\":{\"sides\":[{\"content\":{\"connectorIds\":[\"LConn1\",\"LConn2\"]},\"type\":\"ConnectorPlacement.EquallySpacedRectSide\",\"uuid\":\"35d28eba-fa4f-4cd3-971b-9e32fe878e3c\"},{\"content\":{\"connectorIds\":[\"RConn1\",\"RConn2\",\"RConn3\"],\"side\":\"RIGHT\"},\"type\":\"ConnectorPlacement.EquallySpacedRectSide\",\"uuid\":\"fcb94bdd-c4dd-4816-bcf0-4e4658b36d25\"},{\"content\":{\"connectorIds\":[\"LConn3\"],\"side\":\"TOP\"},\"type\":\"ConnectorPlacement.EquallySpacedRectSide\",\"uuid\":\"9fa0ae4f-ed44-4bac-b091-4976307d3a38\"}]},\"type\":\"ConnectorPlacement.EquallySpacedConnector\",\"uuid\":\"d329ec28-9c00-47af-a114-44f5d27297a5\"}],\"packageUris\":[\"http://schema.mathworks.com/mf0/Connector/R2020b\"],\"version\":\"1.0\"}"
      mask Display: image('Skärmbild 2025-05-02 202341.png');
  Terminator{,1..4} (5 alike) : Terminator
  World Frame : sm_lib/Frames and Transforms/World Frame
  Meas : Outport
  wires:
  Measured Angles/1(Meas) -> Gain/1
  Cmd1/1 -> Cylinder1/1(Cmd)
  Cmd2/1 -> Cylinder2/1(Cmd)
  Gain/1 -> Meas/1
  PS-Simulink Converter/1 -> Radians to Degrees/1
  Radians to Degrees/1 -> Terminator/1  "J4"
  Radians to Degrees1/1 -> Terminator1/1  "J6"
  PS-Simulink Converter1/1 -> Radians to Degrees1/1
  Radians to Degrees2/1 -> Terminator2/1  "J5"
  PS-Simulink Converter2/1 -> Radians to Degrees2/1
  Radians to Degrees3/1 -> Terminator3/1  "J3"
  PS-Simulink Converter3/1 -> Radians to Degrees3/1
  Cmd3/1 -> Cylinder3/1(Cmd)
  PS-Simulink Converter4/1 -> Radians to Degrees4/1
  Radians to Degrees4/1 -> Terminator4/1  "J2"
  connections:
  Pump Speed/RConn1 -- Ideal Angular Velocity Source/RConn1
  Fixed-Displacement Pump (IL)1/RConn1 -- Ideal Angular Velocity Source/LConn1
  Ideal Angular Velocity Source/RConn2 -- Mechanical Rotational Reference/LConn1
  Fixed-Displacement Pump (IL)1/RConn2 -- Mechanical Rotational Reference1/LConn1
  Pressure Relief Valve (IL)/LConn1 -- Constant Volume Chamber (IL)/LConn1 -- Fixed-Displacement Pump (IL)1/LConn1 -- Cylinder1/RConn2 -- Cylinder2/RConn2 -- Cylinder3/RConn2
  Reservoir (IL)/LConn1 -- Fixed-Displacement Pump (IL)1/RConn3 -- Isothermal Liquid Properties (IL)/RConn1 -- Pressure Relief Valve (IL)/RConn1 -- Cylinder1/RConn3 -- Cylinder2/RConn3 -- Cylinder3/RConn3
  J2/LConn1 -- Bom/RConn1
  J3/RConn1 -- Bucket/LConn1
  J4/RConn1 -- LongLinkageArm2/LConn1
  Cylinder2/RConn1 -- Stick/LConn2
  Stick/LConn1 -- J2/RConn1
  Cylinder3/RConn1 -- LinkageArms/LConn2
  Cylinder3/LConn1 -- Stick/RConn3
  Bom/RConn2 -- Cylinder2/LConn1
  J5/LConn1 -- Stick/RConn2
  J6/LConn1 -- LinkageArms/RConn1
  Sensing Angle 1/RConn1 -- Sensing Angle 2/LConn1 -- Bom/LConn3
  Base/LConn2 -- Sensing Angle 1/LConn1
  Base/RConn2 -- Cylinder1/LConn1
  J3/LConn1 -- Stick/RConn1
  J5/RConn1 -- LinkageArms/LConn1
  Bom/LConn1 -- J1/RConn1
  Bucket/LConn2 -- Sensing Angle 3/RConn1
  Cylinder1/RConn1 -- Bom/LConn2
  Stick/LConn3 -- Sensing Angle 2/RConn1 -- Sensing Angle 3/LConn1
  Rigid Transform3/LConn1 -- LongLinkageArm2/RConn1
  J6/RConn1 -- Rigid Transform3/RConn1
  Mechanism Configuration/RConn1 -- Base/LConn1 -- World Frame/RConn1 -- Solver Configuration1/RConn1
  J1/LConn1 -- Base/RConn1
  J4/LConn1 -- Bucket/RConn1
  J4/RConn2 -- PS-Simulink Converter/LConn1
  J6/RConn2 -- PS-Simulink Converter1/LConn1
  J5/RConn2 -- PS-Simulink Converter2/LConn1
  J3/RConn2 -- PS-Simulink Converter3/LConn1
  PS-Simulink Converter4/LConn1 -- J2/RConn2

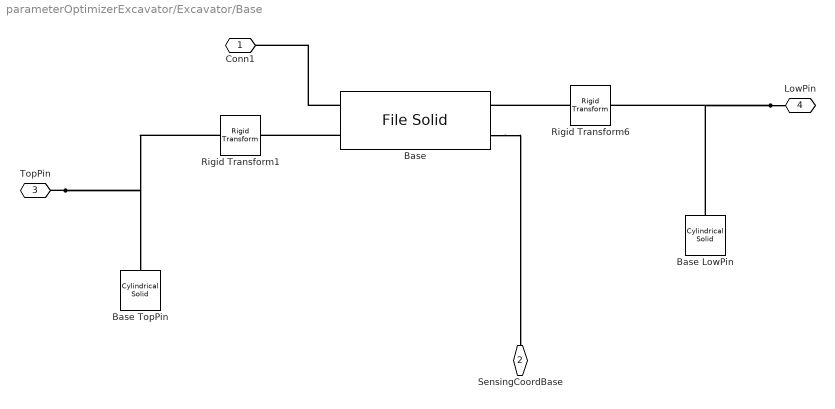
== system parameterOptimizerExcavator/Excavator/Base ==
  Base : sm_lib/Body Elements/File Solid  ExtGeomFileName=CAD/STEPfiles/bas.step  UnitType=Custom  ExtGeomFileUnits=mm  StepReaderType=HEX  ExportConvexHullGeometry=off  InertiaType=CalculateFromGeometry  BasedOnType=Density  Density=1000  DensityUnits=kg/m^3  Mass=1  MassUnits=kg  CenterOfMass=[0 0 0]  CenterOfMassUnits=m  MomentsOfInertia=[1 1 1]  MomentsOfInertiaUnits=kg*m^2  ProductsOfInertia=[0 0 0]  ProductsOfInertiaUnits=kg*m^2  GraphicType=FromGeometry  MarkerShape=Sphere  MarkerSize=10  GraphicVisPropType=SimpleVisualProperties  GraphicDiffuseColor=[0.8 0.8 0.8]  GraphicOpacity=1  GraphicSpecularColor=[0.5 0.5 0.5 1.0]  GraphicAmbientColor=[0.15 0.15 0.15 1.0]  GraphicEmissiveColor=[0.0 0.0 0.0 1.0]  GraphicShininess=75  DoExposeReferenceFrame=off  SerializedFrames=<Frames><Frame><Id>Frame1</Id><Value><Name>BottomCoord</Name><Origin><Source>GeometricFeature</Source><FeatureName>planar surface 34</FeatureName></Origin><PrimaryAxis><DefinedDirection>+Y</DefinedDirection><Source>ReferenceFrame</Source><SourceDirection>+Y</SourceDirection><FeatureName></FeatureName></PrimaryAxis><SecondaryAxis><DefinedDirection>+X</DefinedDirection><Source>ReferenceFrame</Source><SourceDirection>+Z</SourceDirection><FeatureName></FeatureName></SecondaryAxis></Value></Frame><Frame><Id>Frame2</Id><Value><Name>LowerCoord</Name><Origin><Source>GeometricFeature</Source><FeatureName>cylindrical surface 25</FeatureName></Origin><PrimaryAxis><DefinedDirection>+Y</DefinedDirection><Source>ReferenceFrame</Source><SourceDirection>+Y</SourceDirection><FeatureName></FeatureName></PrimaryAxis><SecondaryAxis><DefinedDirection>+X</DefinedDirection><Source>ReferenceFrame</Source><SourceDirection>+Z</SourceDirection><FeatureName></FeatureName></SecondaryAxis></Value></Frame><Frame><Id>Frame3</Id><Value><Name>TopCoord</Name><Origin><Source>GeometricFeature</Source><FeatureName>cylindrical surface 24</FeatureName></Origin><PrimaryAxis><DefinedDirection>+X</DefinedDirection><Source>ReferenceFrame</Source><SourceDirection>+Z</SourceDirection><FeatureName></FeatureName></PrimaryAxis><SecondaryAxis><DefinedDirection>+Y</DefinedDirection><Source>ReferenceFrame</Source><SourceDirection>+Y</SourceDirection><FeatureName></FeatureName></SecondaryAxis></Value></Frame><Frame><Id>Frame4</Id><Value><Name>SensingCoordBase</Name><Origin><Source>GeometricFeature</Source><FeatureName>cylindrical surface 70</FeatureName></Origin><PrimaryAxis><DefinedDirection>+X</DefinedDirection><Source>ReferenceFrame</Source><SourceDirection>+Z</SourceDirection><FeatureName></FeatureName></PrimaryAxis><SecondaryAxis><DefinedDirection>+Y</DefinedDirection><Source>ReferenceFrame</Source><SourceDirection>+Y</SourceDirection><FeatureName></FeatureName></SecondaryAxis></Value></Frame></Frames>
  Base LowPin : sm_lib/Body Elements/Cylindrical Solid  CylinderRadius=Excavator_Param.Link.BaseRadius  CylinderRadiusUnits=m  CylinderLength=Excavator_Param.Link.BaseLength  CylinderLengthUnits=m  ExportEntireGeometry=off  InertiaType=CalculateFromGeometry  BasedOnType=Density  Density=1000  DensityUnits=kg/(m^3)  Mass=1  MassUnits=kg  CenterOfMass=[0 0 0]  CenterOfMassUnits=m  MomentsOfInertia=[1 1 1]  MomentsOfInertiaUnits=kg*m^2  ProductsOfInertia=[0 0 0]  ProductsOfInertiaUnits=kg*m^2  GraphicType=FromGeometry  MarkerShape=Sphere  MarkerSize=10  GraphicVisPropType=SimpleVisualProperties  GraphicDiffuseColor=[0.149 0.149 0.149]  GraphicOpacity=1.0  GraphicSpecularColor=[0.5 0.5 0.5 1.0]  GraphicAmbientColor=[0.15 0.15 0.15 1.0]  GraphicEmissiveColor=[0.0 0.0 0.0 1.0]  GraphicShininess=75  DoExposeReferenceFrame=on  SerializedFrames=<Frames/>
  Base TopPin : sm_lib/Body Elements/Cylindrical Solid  CylinderRadius=Excavator_Param.Link.BaseRadius  CylinderRadiusUnits=m  CylinderLength=Excavator_Param.Link.BaseLength  CylinderLengthUnits=m  ExportEntireGeometry=off  InertiaType=CalculateFromGeometry  BasedOnType=Density  Density=1000  DensityUnits=kg/(m^3)  Mass=1  MassUnits=kg  CenterOfMass=[0 0 0]  CenterOfMassUnits=m  MomentsOfInertia=[1 1 1]  MomentsOfInertiaUnits=kg*m^2  ProductsOfInertia=[0 0 0]  ProductsOfInertiaUnits=kg*m^2  GraphicType=FromGeometry  MarkerShape=Sphere  MarkerSize=10  GraphicVisPropType=SimpleVisualProperties  GraphicDiffuseColor=[0.149 0.149 0.149]  GraphicOpacity=1.0  GraphicSpecularColor=[0.5 0.5 0.5 1.0]  GraphicAmbientColor=[0.15 0.15 0.15 1.0]  GraphicEmissiveColor=[0.0 0.0 0.0 1.0]  GraphicShininess=75  DoExposeReferenceFrame=on  SerializedFrames=<Frames/>
  Rigid Transform1 : sm_lib/Frames and Transforms/Rigid Transform  RotationMethod=None  FollAlignAxisA=+X  BaseAlignAxisA=+Y  FollAlignAxisB=+Y  BaseAlignAxisB=+Z  RotationStandardAxis=+Z  RotationAngle=0  RotationAngleUnits=deg  RotationArbitraryAxis=[0 0 1]  RotationSequenceAxes=FollowerAxes  RotationSequence=XYX  RotationSequenceAngles=[0 0 0]  RotationSequenceAnglesUnits=deg  RotationMatrix=[1 0 0;0 1 0;0 0 1]  Quaternion=[1 0 0 0]  TranslationMethod=StandardAxis  TranslationCartesianOffset=[0 0 0]  TranslationCartesianOffsetUnits=m  TranslationStandardAxis=+Z  TranslationStandardOffset=(Excavator_Param.Base.InnerWidth/2) + (Excavator_Param.Base.CutoutWidth/2)  TranslationStandardOffsetUnits=m  TranslationROffset=0  TranslationROffsetUnits=m  TranslationThetaOffset=0  TranslationThetaOffsetUnits=deg  TranslationZOffset=0  TranslationZOffsetUnits=m
  Rigid Transform6 : sm_lib/Frames and Transforms/Rigid Transform  RotationMethod=None  FollAlignAxisA=+X  BaseAlignAxisA=+Y  FollAlignAxisB=+Y  BaseAlignAxisB=+Z  RotationStandardAxis=+Z  RotationAngle=0  RotationAngleUnits=deg  RotationArbitraryAxis=[0 0 1]  RotationSequenceAxes=FollowerAxes  RotationSequence=XYX  RotationSequenceAngles=[0 0 0]  RotationSequenceAnglesUnits=deg  RotationMatrix=[1 0 0;0 1 0;0 0 1]  Quaternion=[1 0 0 0]  TranslationMethod=StandardAxis  TranslationCartesianOffset=[0 0 0]  TranslationCartesianOffsetUnits=m  TranslationStandardAxis=+Z  TranslationStandardOffset=(Excavator_Param.Base.InnerWidth/2) + (Excavator_Param.Base.CutoutWidth/2)  TranslationStandardOffsetUnits=m  TranslationROffset=0  TranslationROffsetUnits=m  TranslationThetaOffset=0  TranslationThetaOffsetUnits=deg  TranslationZOffset=0  TranslationZOffsetUnits=m
  Conn1 : PMIOPort  Side=Left
  SensingCoordBase : PMIOPort  Port=2  Side=Left
  TopPin : PMIOPort  Port=3  Side=Right
  LowPin : PMIOPort  Port=4  Side=Right
  connections:
  Base/RConn2 -- SensingCoordBase/RConn1
  Base/LConn2 -- Rigid Transform1/LConn1
  LowPin/RConn1 -- Rigid Transform6/RConn1 -- Base LowPin/RConn1
  Rigid Transform6/LConn1 -- Base/RConn1
  Base/LConn1 -- Conn1/RConn1
  TopPin/RConn1 -- Base TopPin/RConn1 -- Rigid Transform1/RConn1
